simulink model "HW2_es2"  (R2024a)
settings: Solver=VariableStepAuto  StartTime=0.0  StopTime=Tsca  RelTol=1e-3
values from neighbouring files (symbols this model uses):
  b = load('ERROR_NORM_0.1.mat')    [H2.m]
  k1 = 5    [H2.m]
  k2 = 5    [H2.m]
libraries: robotmobilelib x1
settings Model: Creator=Strix  LastModifiedBy=Strix

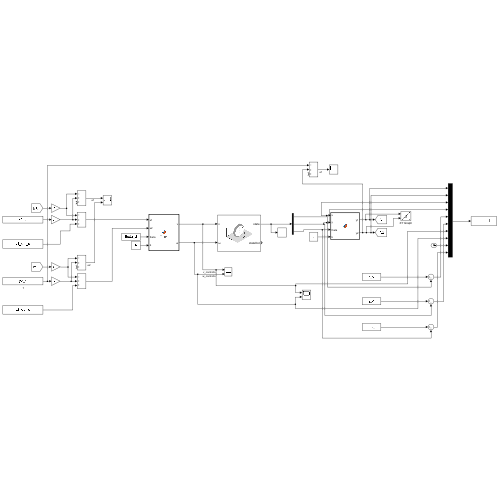
[thumbnail: Simulink's stored preview of the top-level diagram]
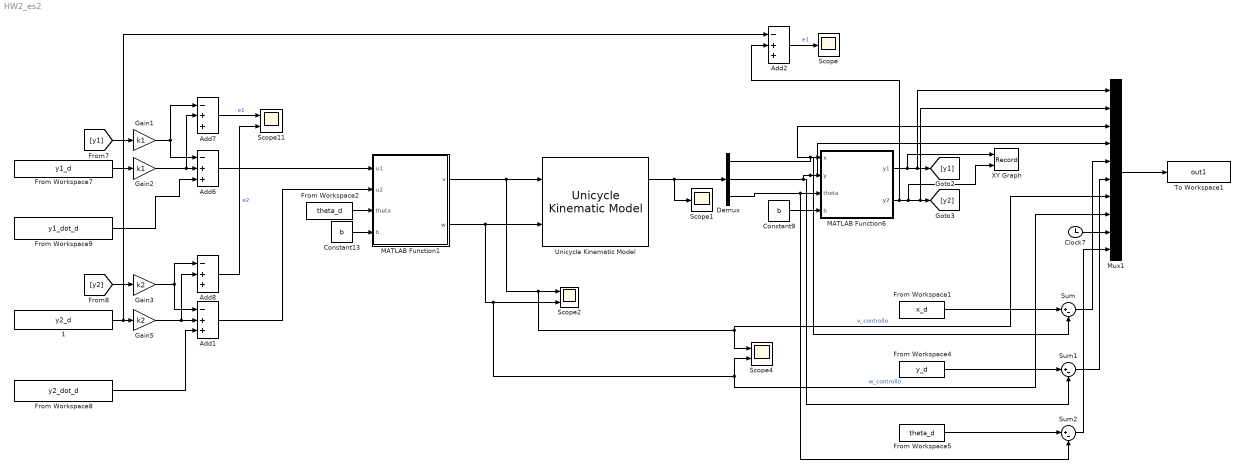
== system HW2_es2 ==
  " 1" : FromWorkspace  VariableName=y2_d
  Add{1..2,6..8} (5 alike) : Sum  Inputs=-++
  Clock7 : Clock
  Constant13 : Constant  Value=b
  Constant9 : Constant  Value=b
  Demux : Demux  Outputs=3
  From Workspace1 : FromWorkspace  VariableName=x_d
  From Workspace2 : FromWorkspace  VariableName=theta_d
  From Workspace4 : FromWorkspace  VariableName=y_d
  From Workspace5 : FromWorkspace  VariableName=theta_d
  From Workspace7 : FromWorkspace  VariableName=y1_d
  From Workspace8 : FromWorkspace  VariableName=y2_dot_d
  From Workspace9 : FromWorkspace  VariableName=y1_dot_d
  Gain1 : Gain  Gain=k1
  Gain2 : Gain  Gain=k1
  Gain3 : Gain  Gain=k2
  Gain5 : Gain  Gain=k2
  MATLAB Function1 : MATLAB Function  TreatAsAtomicUnit=on
  MATLAB Function6 : MATLAB Function  TreatAsAtomicUnit=on
  Mux1 : Mux  Inputs=10
  Scope : Scope
  Scope1 : Scope
  Scope11 : Scope  NumInputPorts=2
  Scope2 : Scope  NumInputPorts=2
  Scope4 : Scope  NumInputPorts=2
  Sum : Sum  Inputs=|+-
  Sum1 : Sum  Inputs=|+-
  Sum2 : Sum  Inputs=|+-
  To Workspace1 : ToWorkspace  VariableName=out1  SampleTime=-1
  Unicycle Kinematic Model : robotmobilelib/Unicycle Kinematic Model  VehicleInputs=Vehicle Speed & Heading Angular Velocity  WheelRadius=0.1  WheelSpeedRange=[-Inf Inf]  InitialState=[0; 0; 0]  SimulateUsing=Interpreted execution
  XY Graph : Record  FileSettingsInternal="{\"entries\":[{\"content\":{\"excelSettings\":{\"content\":{},\"type\":\"Streamout.ExcelSettings\"}},\"type\":\"Streamout.FileSettingStorage\",\"uuid\":\"\"}],\"packageUris\":[\"http:\\/\\/schema.mathworks.com\\/mf0\\/streamout_blocks\\/R2020a\"],\"version\":\"1.0\"}"  Layout=[1 1]  SignalsInternal="{\"entries\":[{\"content\":{\"signals\":[{\"content\":{\"blockPath\":[],\"dimensions\":[1],\"domain\":\"\",\"lineColor\":\"#a2142f\",\"plots\":[ 1 ],\"port\":1,\"sid\":[\"\"],\"signalID\":1,\"signalName\":\"MATLAB Function6:1\"},\"type\":\"RecordBlkView.Signal\",\"uuid\":\"\"},{\"content\":{\"blockPath\":[],\"dimensions\":[1],\"domain\":\"\",\"lineColor\":\"#139fff\",\"plots\":[ 1 ],\"port\":2,\"sid\":[\"\"],\"signalID\":2,\"signalName\":\"MATLAB Function6:2\"},\"type\":\"RecordBlkView.Signal\",\"uuid\":\"\"}]},\"type\":\"RecordBlkView.InputSignals\",\"uuid\":\"\"}],\"packageUris\":[\"http:\\/\\/schema.mathworks.com\\/mf0\\/streamout_blocks\\/R2020a\"],\"version\":\"1.0\"}"  VisualizationBindings="{\"xyplotplugin\":{\"info\":[{\"series\":[{\"bindingParametersList\":[{\"parameter\":\"X-Axis\",\"signalID\":1,\"signalName\":\"MATLAB Function6:1\"},{\"parameter\":\"Y-Axis\",\"signalID\":2,\"signalName\":\"MATLAB Function6:2\"}],\"seriesID\":0}],\"subplotID\":1}]}}"  CompatibilityTag=XY
  wires:
  From Workspace8/1 -> Add1/3
  " 1"/1 -> Add2/1, Gain5/1
  Gain1/1 -> Add7/1, Add6/1
  Clock7/1 -> Mux1/9
  Gain2/1 -> Add7/2, Add6/2
  Add8/1 -> Scope11/2  "e2"
  [y2] -> Gain3/1
  [y1] -> Gain1/1
  MATLAB Function6/2(y2) -> Add2/2, XY Graph/2, Mux1/2, [y2]
  MATLAB Function6/1(y1) -> XY Graph/1, Mux1/1, [y1]
  Demux/2 -> Sum1/2, Mux1/4, MATLAB Function6/2(y)
  Unicycle Kinematic Model/1 -> Demux/1, Scope1/1
  Demux/1 -> Sum/2, Mux1/3, MATLAB Function6/1(x)
  Sum/1 -> Mux1/5
  Sum2/1 -> Mux1/10
  From Workspace5/1 -> Sum2/1
  From Workspace1/1 -> Sum/1
  Demux/3 -> Sum2/2, MATLAB Function6/3(theta)
  Add7/1 -> Scope11/1  "e1"
  From Workspace9/1 -> Add6/3
  From Workspace4/1 -> Sum1/1
  Add1/1 -> MATLAB Function1/2(u2)
  Constant9/1 -> MATLAB Function6/4(b)
  Mux1/1 -> To Workspace1/1
  Constant13/1 -> MATLAB Function1/4(b)
  MATLAB Function1/2(w) -> Mux1/8, Scope4/2, Scope2/2, Unicycle Kinematic Model/2  "w_controllo"
  MATLAB Function1/1(v) -> Unicycle Kinematic Model/1, Scope4/1, Mux1/7, Scope2/1  "v_controllo"
  Gain5/1 -> Add1/2, Add8/2
  Gain3/1 -> Add8/1, Add1/1
  From Workspace7/1 -> Gain2/1
  Add6/1 -> MATLAB Function1/1(u1)
  Add2/1 -> Scope/1  "e1"
  Sum1/1 -> Mux1/6
  From Workspace2/1 -> MATLAB Function1/3(theta)

== matlab function HW2_es2/MATLAB Function1 ==
  data: u1 input; v output; u2 input; theta input; w output; b input
function [v,w] = T_inv(u1,u2,theta,b)

T=[cos(theta)  -b*sin(theta)
    sin(theta)  b*cos(theta)];

vw = inv(T) * [u1; u2];  % usa ; oppure [u1 u2]' per colonna
v  = vw(1);
w  = vw(2);
end

== matlab function HW2_es2/MATLAB Function6 ==
  data: x input; y1 output; y input; theta input; y2 output; b input
function [y1 , y2] = T(x,y,theta,b)

y1 = x + b*cos(theta);
y2 = y + b*sin(theta);

end
